simulink library "BeamNG_interface"  (R2022b)
settings: Solver=VariableStepAuto  StartTime=0.0  StopTime=10.0  RelTol=1e-3
libraries: $bdroot x1
settings Model: Creator=matti  LastModifiedBy=matti

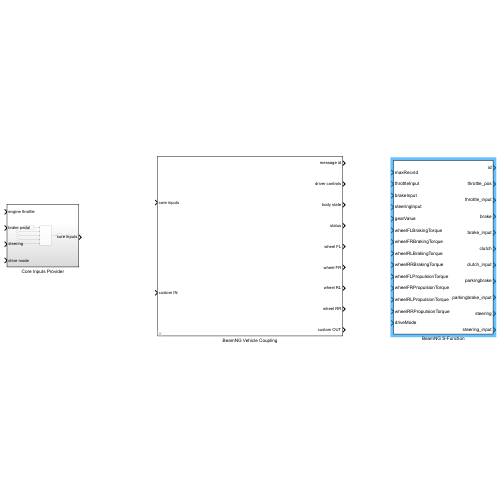
[thumbnail: Simulink's stored preview of the top-level diagram]
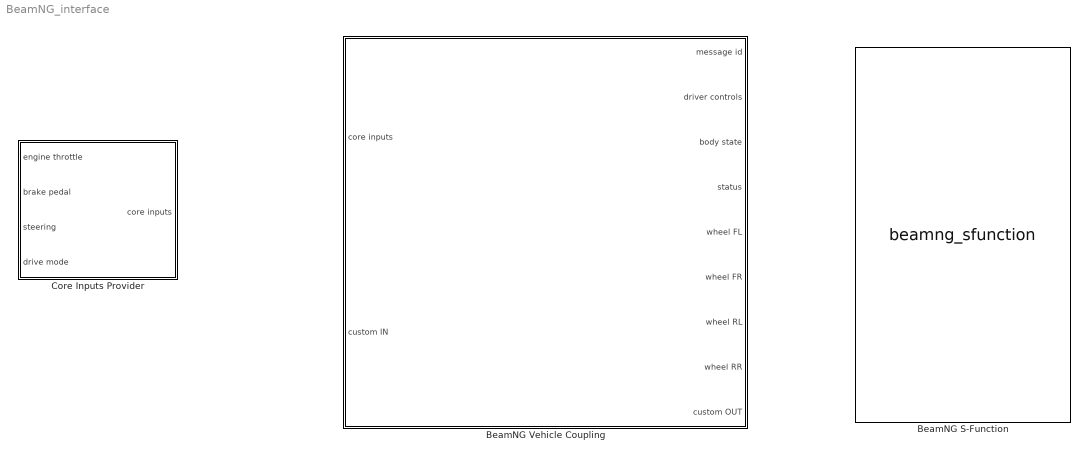
== system BeamNG_interface ==
  BeamNG S-Function : S-Function  FunctionName=beamng_sfunction  Parameters=64890, 64891, '127.0.0.1', '127.0.0.1', 'C:\Users\matti\Downloads\signals_list.csv'  SFunctionDeploymentMode=off  EnableBusSupport=off
      mask Display:
      | handles = get_param(gcb, "PortHandles");
      | num_inputs = length(handles.Inport);
      | num_outputs = length(handles.Outport);
      | 
      | params = get_param(gcb, "Parameters");
      | pattern = '''(.*?)''';
      | params = regexp(params, pattern, 'tokens');
      | csv_path = params{3}{1};
      | 
      | T = readtable(csv_path);
      | 
      | input_labels = cell(num_inputs, 1);
      | output_labels = cell(num_outputs, 1);
      | 
      | in = 1;
      | out = 1;
      | 
      | for i = 1:height(T)
      |     direction = T{i, 4}{1};
      |     if strcmp(direction, 'BeamNG_to_Simulink')
      |         output_labels{out} = T{i, 3}{1};
      |         out = out + 1;
      |     elseif strcmp(direction, 'Simulink_to_BeamNG')
      |         input_labels{in} = T{i, 3}{1};
      |         in = in + 1;
      |     end
      | end
      | 
      | for i = 1:num_inputs
      |     port_label('input', i, input_labels{i})
      | end
      | 
      | for i = 1:num_outputs
      |     port_label('output', i, output_labels{i})
      | end
  BeamNG Vehicle Coupling : Subsystem  mask(BeamNG Vehicle Coupling){}
      mask help: This block is a more handy interface for the BeamNG S-Function
      mask Help: Output as buses
  Core Inputs Provider : Subsystem

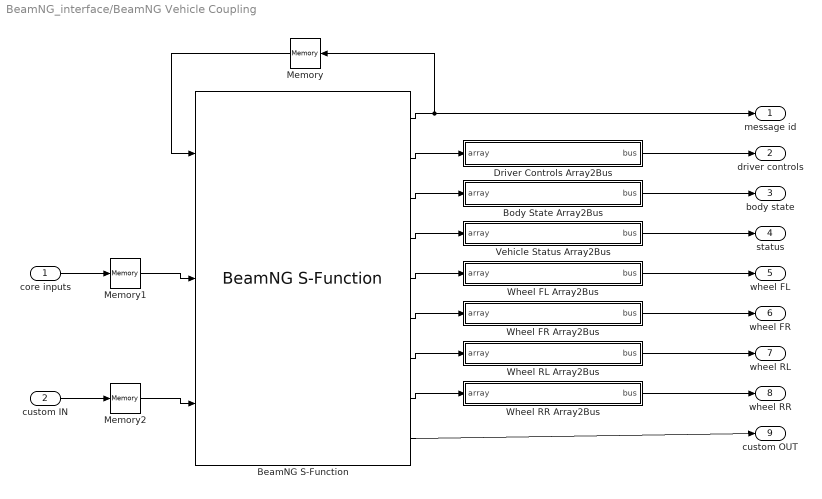
== system BeamNG_interface/BeamNG Vehicle Coupling ==
  core inputs : Inport
  custom IN : Inport  Port=2
  BeamNG S-Function : $bdroot/BeamNG S-Function  SFunctionModules=''
  Body State Array2Bus : Subsystem
  Driver Controls Array2Bus : Subsystem
  Memory : Memory
  Memory1 : Memory
  Memory2 : Memory
  Vehicle Status Array2Bus : Subsystem
  Wheel FL Array2Bus : Subsystem
  Wheel FR Array2Bus : Subsystem
  Wheel RL Array2Bus : Subsystem
  Wheel RR Array2Bus : Subsystem
  message id : Outport
  driver controls : Outport  Port=2
  body state : Outport  Port=3
  status : Outport  Port=4
  wheel FL : Outport  Port=5
  wheel FR : Outport  Port=6
  wheel RL : Outport  Port=7
  wheel RR : Outport  Port=8
  custom OUT : Outport  Port=9
  wires:
  BeamNG S-Function/6 -> Wheel FR Array2Bus/1(array)
  BeamNG S-Function/3 -> Body State Array2Bus/1(array)
  Memory/1 -> BeamNG S-Function/1
  BeamNG S-Function/1 -> message id/1, Memory/1
  BeamNG S-Function/7 -> Wheel RL Array2Bus/1(array)
  BeamNG S-Function/4 -> Vehicle Status Array2Bus/1(array)
  BeamNG S-Function/5 -> Wheel FL Array2Bus/1(array)
  BeamNG S-Function/8 -> Wheel RR Array2Bus/1(array)
  custom IN/1 -> Memory2/1
  Driver Controls Array2Bus/1(bus) -> driver controls/1
  BeamNG S-Function/2 -> Driver Controls Array2Bus/1(array)
  Body State Array2Bus/1(bus) -> body state/1
  BeamNG S-Function/9 -> custom OUT/1
  core inputs/1 -> Memory1/1
  Vehicle Status Array2Bus/1(bus) -> status/1
  Wheel FL Array2Bus/1(bus) -> wheel FL/1
  Wheel FR Array2Bus/1(bus) -> wheel FR/1
  Wheel RL Array2Bus/1(bus) -> wheel RL/1
  Wheel RR Array2Bus/1(bus) -> wheel RR/1
  Memory1/1 -> BeamNG S-Function/2
  Memory2/1 -> BeamNG S-Function/3

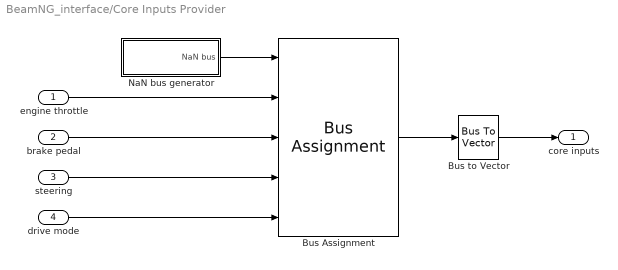
== system BeamNG_interface/Core Inputs Provider ==
  engine throttle : Inport
  brake pedal : Inport  Port=2
  steering : Inport  Port=3
  drive mode : Inport  Port=4
  Bus Assignment : BusAssignment  AssignedSignals=engine throttle,brake pedal,steering,drive mode
  Bus to Vector : BusToVector
  NaN bus generator : Subsystem
  core inputs : Outport
  wires:
  NaN bus generator/1(NaN bus) -> Bus Assignment/1
  Bus Assignment/1 -> Bus to Vector/1
  drive mode/1 -> Bus Assignment/5
  engine throttle/1 -> Bus Assignment/2
  Bus to Vector/1 -> core inputs/1
  steering/1 -> Bus Assignment/4
  brake pedal/1 -> Bus Assignment/3

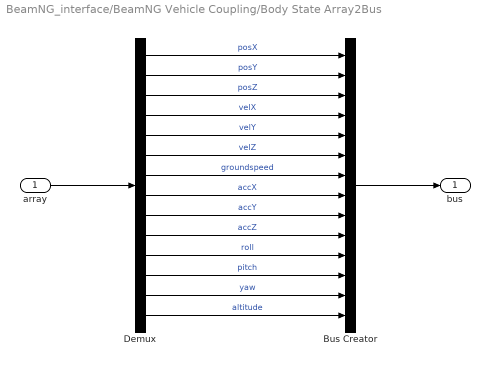
== system BeamNG_interface/BeamNG Vehicle Coupling/Body State Array2Bus ==
  array : Inport
  Bus Creator : BusCreator  Inputs=14
  Demux : Demux  Outputs=14
  bus : Outport
  wires:
  Bus Creator/1 -> bus/1
  array/1 -> Demux/1
  Demux/14 -> Bus Creator/14  "altitude"
  Demux/13 -> Bus Creator/13  "yaw"
  Demux/12 -> Bus Creator/12  "pitch"
  Demux/11 -> Bus Creator/11  "roll"
  Demux/10 -> Bus Creator/10  "accZ"
  Demux/9 -> Bus Creator/9  "accY"
  Demux/8 -> Bus Creator/8  "accX"
  Demux/7 -> Bus Creator/7  "groundspeed"
  Demux/6 -> Bus Creator/6  "velZ"
  Demux/5 -> Bus Creator/5  "velY"
  Demux/4 -> Bus Creator/4  "velX"
  Demux/3 -> Bus Creator/3  "posZ"
  Demux/2 -> Bus Creator/2  "posY"
  Demux/1 -> Bus Creator/1  "posX"

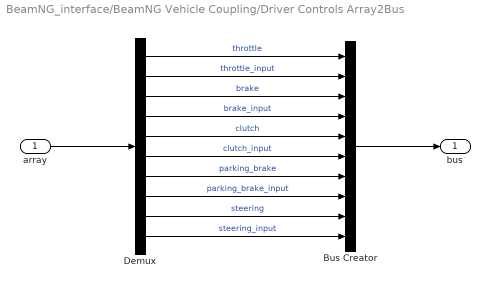
== system BeamNG_interface/BeamNG Vehicle Coupling/Driver Controls Array2Bus ==
  array : Inport
  Bus Creator : BusCreator  Inputs=10
  Demux : Demux  Outputs=10
  bus : Outport
  wires:
  Demux/2 -> Bus Creator/2  "throttle_input"
  Demux/1 -> Bus Creator/1  "throttle"
  array/1 -> Demux/1
  Bus Creator/1 -> bus/1
  Demux/3 -> Bus Creator/3  "brake"
  Demux/4 -> Bus Creator/4  "brake_input"
  Demux/5 -> Bus Creator/5  "clutch"
  Demux/6 -> Bus Creator/6  "clutch_input"
  Demux/7 -> Bus Creator/7  "parking_brake"
  Demux/8 -> Bus Creator/8  "parking_brake_input"
  Demux/9 -> Bus Creator/9  "steering"
  Demux/10 -> Bus Creator/10  "steering_input"

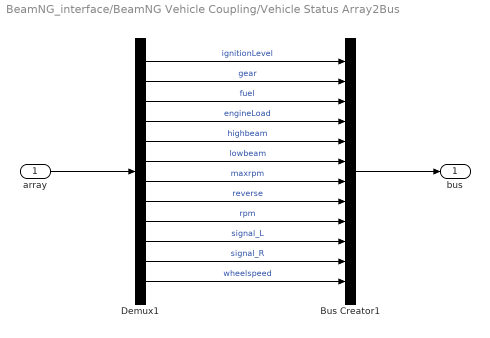
== system BeamNG_interface/BeamNG Vehicle Coupling/Vehicle Status Array2Bus ==
  array : Inport
  Bus Creator1 : BusCreator  Inputs=12
  Demux1 : Demux  Outputs=12
  bus : Outport
  wires:
  array/1 -> Demux1/1
  Bus Creator1/1 -> bus/1
  Demux1/1 -> Bus Creator1/1  "ignitionLevel"
  Demux1/2 -> Bus Creator1/2  "gear"
  Demux1/3 -> Bus Creator1/3  "fuel"
  Demux1/5 -> Bus Creator1/5  "highbeam"
  Demux1/4 -> Bus Creator1/4  "engineLoad"
  Demux1/6 -> Bus Creator1/6  "lowbeam"
  Demux1/7 -> Bus Creator1/7  "maxrpm"
  Demux1/8 -> Bus Creator1/8  "reverse"
  Demux1/9 -> Bus Creator1/9  "rpm"
  Demux1/10 -> Bus Creator1/10  "signal_L"
  Demux1/11 -> Bus Creator1/11  "signal_R"
  Demux1/12 -> Bus Creator1/12  "wheelspeed"

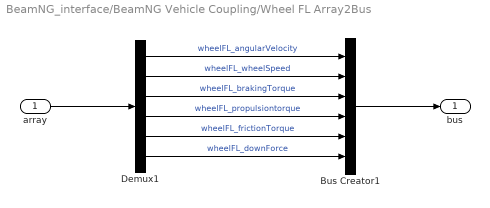
== system BeamNG_interface/BeamNG Vehicle Coupling/Wheel FL Array2Bus ==
  array : Inport
  Bus Creator1 : BusCreator  Inputs=6
  Demux1 : Demux  Outputs=6
  bus : Outport
  wires:
  array/1 -> Demux1/1
  Bus Creator1/1 -> bus/1
  Demux1/1 -> Bus Creator1/1  "wheelFL_angularVelocity"
  Demux1/2 -> Bus Creator1/2  "wheelFL_wheelSpeed"
  Demux1/3 -> Bus Creator1/3  "wheelFL_brakingTorque"
  Demux1/4 -> Bus Creator1/4  "wheelFL_propulsiontorque"
  Demux1/5 -> Bus Creator1/5  "wheelFL_frictionTorque"
  Demux1/6 -> Bus Creator1/6  "wheelFL_downForce"

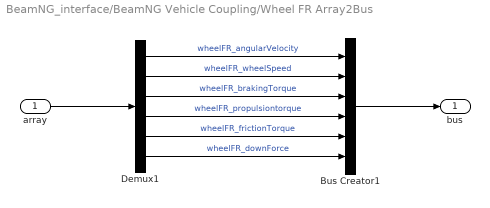
== system BeamNG_interface/BeamNG Vehicle Coupling/Wheel FR Array2Bus ==
  array : Inport
  Bus Creator1 : BusCreator  Inputs=6
  Demux1 : Demux  Outputs=6
  bus : Outport
  wires:
  Demux1/6 -> Bus Creator1/6  "wheelFR_downForce"
  Demux1/5 -> Bus Creator1/5  "wheelFR_frictionTorque"
  Demux1/4 -> Bus Creator1/4  "wheelFR_propulsiontorque"
  Demux1/3 -> Bus Creator1/3  "wheelFR_brakingTorque"
  Demux1/2 -> Bus Creator1/2  "wheelFR_wheelSpeed"
  Demux1/1 -> Bus Creator1/1  "wheelFR_angularVelocity"
  Bus Creator1/1 -> bus/1
  array/1 -> Demux1/1

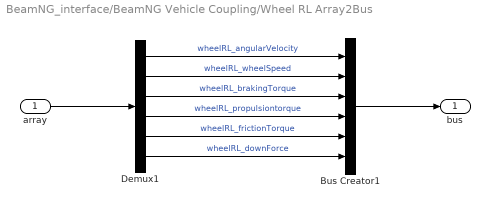
== system BeamNG_interface/BeamNG Vehicle Coupling/Wheel RL Array2Bus ==
  array : Inport
  Bus Creator1 : BusCreator  Inputs=6
  Demux1 : Demux  Outputs=6
  bus : Outport
  wires:
  array/1 -> Demux1/1
  Bus Creator1/1 -> bus/1
  Demux1/1 -> Bus Creator1/1  "wheelRL_angularVelocity"
  Demux1/2 -> Bus Creator1/2  "wheelRL_wheelSpeed"
  Demux1/3 -> Bus Creator1/3  "wheelRL_brakingTorque"
  Demux1/4 -> Bus Creator1/4  "wheelRL_propulsiontorque"
  Demux1/5 -> Bus Creator1/5  "wheelRL_frictionTorque"
  Demux1/6 -> Bus Creator1/6  "wheelRL_downForce"

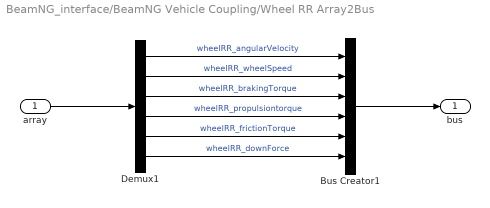
== system BeamNG_interface/BeamNG Vehicle Coupling/Wheel RR Array2Bus ==
  array : Inport
  Bus Creator1 : BusCreator  Inputs=6
  Demux1 : Demux  Outputs=6
  bus : Outport
  wires:
  Demux1/6 -> Bus Creator1/6  "wheelRR_downForce"
  Demux1/5 -> Bus Creator1/5  "wheelRR_frictionTorque"
  Demux1/4 -> Bus Creator1/4  "wheelRR_propulsiontorque"
  Demux1/3 -> Bus Creator1/3  "wheelRR_brakingTorque"
  Demux1/2 -> Bus Creator1/2  "wheelRR_wheelSpeed"
  Demux1/1 -> Bus Creator1/1  "wheelRR_angularVelocity"
  Bus Creator1/1 -> bus/1
  array/1 -> Demux1/1

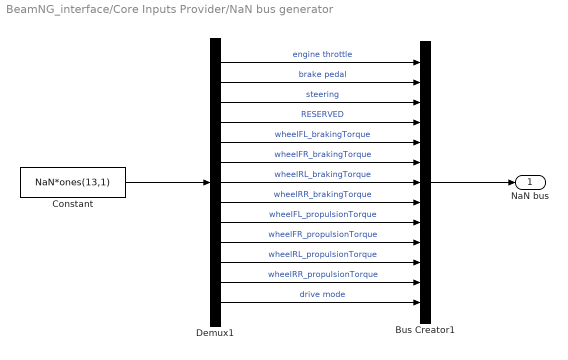
== system BeamNG_interface/Core Inputs Provider/NaN bus generator ==
  Bus Creator1 : BusCreator  Inputs=13
  Constant : Constant  Value=NaN*ones(13,1)
  Demux1 : Demux  Outputs=13
  NaN bus : Outport
  wires:
  Bus Creator1/1 -> NaN bus/1
  Demux1/13 -> Bus Creator1/13  "drive mode"
  Demux1/12 -> Bus Creator1/12  "wheelRR_propulsionTorque"
  Demux1/11 -> Bus Creator1/11  "wheelRL_propulsionTorque"
  Demux1/10 -> Bus Creator1/10  "wheelFR_propulsionTorque"
  Demux1/9 -> Bus Creator1/9  "wheelFL_propulsionTorque"
  Demux1/8 -> Bus Creator1/8  "wheelRR_brakingTorque"
  Demux1/7 -> Bus Creator1/7  "wheelRL_brakingTorque"
  Demux1/6 -> Bus Creator1/6  "wheelFR_brakingTorque"
  Demux1/5 -> Bus Creator1/5  "wheelFL_brakingTorque"
  Demux1/4 -> Bus Creator1/4  "RESERVED"
  Demux1/3 -> Bus Creator1/3  "steering"
  Demux1/2 -> Bus Creator1/2  "brake pedal"
  Demux1/1 -> Bus Creator1/1  "engine throttle"
  Constant/1 -> Demux1/1
